simulink model "gabs_block_diagram"  (R2023a)
settings: Solver=VariableStepAuto  StartTime=0.0  StopTime=10.0  RelTol=1e-3
settings Model: Creator=pinki  LastModifiedBy=pinki

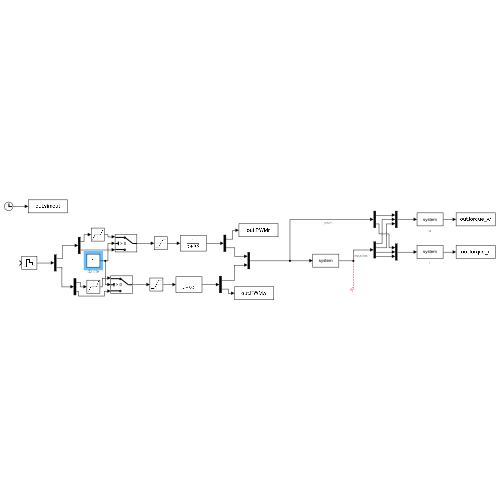
[thumbnail: Simulink's stored preview of the top-level diagram]
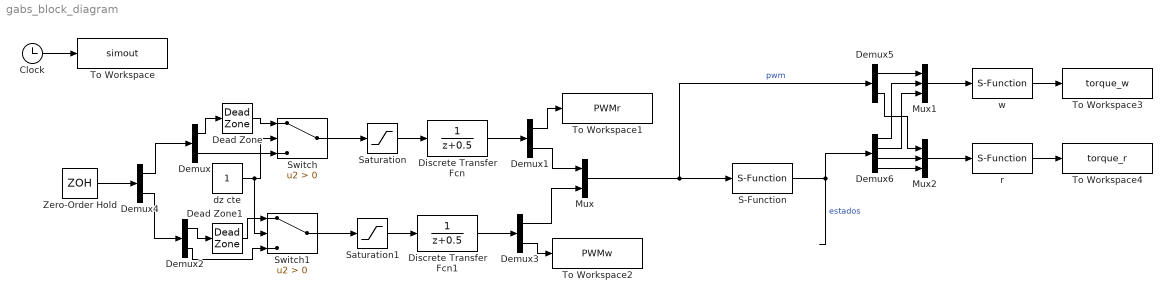
== system gabs_block_diagram ==
  Clock : Clock
  Dead Zone : DeadZone
  Dead Zone1 : DeadZone
  Demux{,1..5} (6 alike) : Demux  Outputs=2
  Demux6 : Demux
  Discrete Transfer Fcn : DiscreteTransferFcn
  Discrete Transfer Fcn1 : DiscreteTransferFcn
  Mux : Mux  Inputs=2
  Mux1 : Mux  Inputs=3
  Mux2 : Mux  Inputs=3
  S-Function : S-Function  SFunctionDeploymentMode=off  EnableBusSupport=off
  Saturation : Saturate
  Saturation1 : Saturate
  Switch : Switch  Criteria=u2 > Threshold  SaturateOnIntegerOverflow=off  InputSameDT=off
  Switch1 : Switch  Criteria=u2 > Threshold  SaturateOnIntegerOverflow=off  InputSameDT=off
  To Workspace : ToWorkspace  VariableName=simout  SaveFormat=Timeseries  SampleTime=-1
  To Workspace1 : ToWorkspace  VariableName=PWMr  SaveFormat=Timeseries  SampleTime=-1
  To Workspace2 : ToWorkspace  VariableName=PWMw  SaveFormat=Timeseries  SampleTime=-1
  To Workspace3 : ToWorkspace  VariableName=torque_w  SaveFormat=Timeseries  SampleTime=-1
  To Workspace4 : ToWorkspace  VariableName=torque_r  SaveFormat=Timeseries  SampleTime=-1
  Zero-Order Hold : ZeroOrderHold  SampleTime=-1
  dz cte : Constant
  r : S-Function  SFunctionDeploymentMode=off  EnableBusSupport=off
  w : S-Function  SFunctionDeploymentMode=off  EnableBusSupport=off
  wires:
  Clock/1 -> To Workspace/1
  Demux4/1 -> Demux/1
  Demux/1 -> Dead Zone/1
  Dead Zone/1 -> Switch/1
  Demux/2 -> Switch/3
  dz cte/1 -> Switch/2, Switch1/2
  Switch/1 -> Saturation/1
  Saturation/1 -> Discrete Transfer Fcn/1
  Discrete Transfer Fcn/1 -> Demux1/1
  Demux1/1 -> To Workspace1/1
  Demux1/2 -> Mux/1
  Discrete Transfer Fcn1/1 -> Demux3/1
  Switch1/1 -> Saturation1/1
  Demux2/1 -> Dead Zone1/1
  Demux2/2 -> Switch1/3
  Demux4/2 -> Demux2/1
  Demux3/2 -> To Workspace2/1
  Dead Zone1/1 -> Switch1/1
  Saturation1/1 -> Discrete Transfer Fcn1/1
  Demux3/1 -> Mux/2
  Zero-Order Hold/1 -> Demux4/1
  Mux/1 -> Demux5/1, S-Function/1  "pwm"
  Demux5/1 -> Mux1/1
  Mux1/1 -> w/1
  w/1 -> To Workspace3/1
  S-Function/1 -> Demux6/1  "estados"
  Demux6/1 -> Mux1/2
  Demux6/2 -> Mux1/3
  Mux2/1 -> r/1
  Demux6/3 -> Mux2/2
  Demux6/4 -> Mux2/3
  Demux5/2 -> Mux2/1
  r/1 -> To Workspace4/1
